simulink model "SG__MDL_IO104_VirtualShift"  (R2022a)
settings: Solver=FixedStepAuto  StartTime=0.0  StopTime=Inf  RelTol=1e-3  EnableMultiTasking=on
model workspace (MAT data in the model file):
  a = 0.28
  ff = 1200
  fi = 150
  tmax = 40
undefined symbols (not defined in the file or in its folder): Ended, Single
libraries: simulink x4, speedgoatlib_IO104 x3, hdlsllib x2, slrealtimeloglib x1, dspsrcs4 x1
settings Model: SimulationMode=external  Creator=padlewsk  LastModifiedBy=padlewsk
settings SolverCC: ConcurrentTasks=on  AlgebraicLoopSolver=TrustRegion  PositivePriorityOrder=on  AutoInsertRateTranBlk=on
settings DataIOCC: SaveFormat=StructureWithTime
settings OptimizationCC: BlockReduction=off  OptimizeBlockIOStorage=off
settings DebuggingCC: TasksWithSamePriorityMsg=none  UnconnectedInputMsg=warning  UnconnectedOutputMsg=warning  UnconnectedLineMsg=warning
settings HardwareCC: ProdBitPerLong=64  ProdLongLongMode=on  ProdHWDeviceType=Intel->x86-64 (Linux 64)
settings RTWCC: Description=Simulink Real-Time  SystemTargetFile=slrealtime.tlc  TemplateMakefile=slrealtime_default_tmf  Toolchain=Simulink Real-Time Toolchain  BuildConfiguration=Faster Runs  CodeExecutionProfiling=on  TargetLang=C++

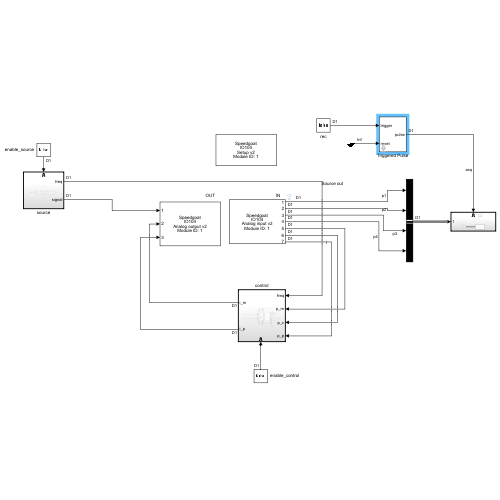
[thumbnail: Simulink's stored preview of the top-level diagram]
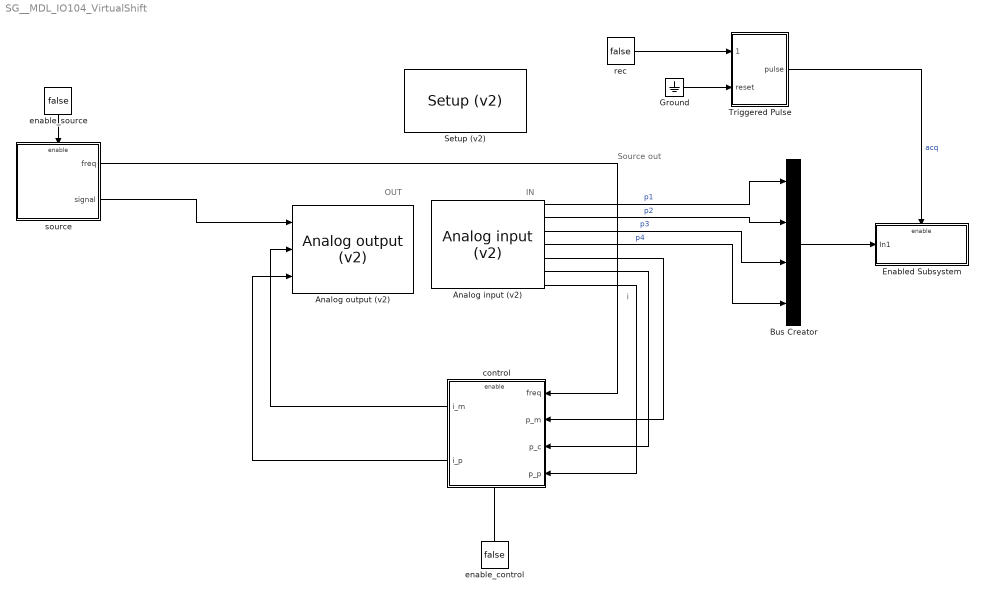
== system SG__MDL_IO104_VirtualShift ==
  note: i
  note: Source out
  note: IN
  note: OUT
  "Analog input (v2) " : speedgoatlib_IO104/Analog input (v2)   parModuleId=1  parTs=-1  parPciSlot=-1  parAdChannels=[1,2,3,4,5,6,7]  parAdChannelsSorted=[1,2,3,4,5,6,7]  parAdRange1=+-10V  parAdRange2=+-10V  parAdCoupling=Single-Ended  parAdFrameSize=1  parAdUseTrigger=off  parAdClockInitiator=Initiator  parAdSampleTime=9.920634921e-07  parTriggerInitiator=Target  parTriggerRate=4.161015625e-01
      settings: SourceProductName=Simulink Real-Time: Speedgoat I/O Blockset
  "Analog output (v2) " : speedgoatlib_IO104/Analog output (v2)   parModuleId=1  parTs=-1  parPciSlot=-1  parDaChannels=[1,2,3]  parDaChannelsSorted=[1,2,3]  parDaInitValue=[0,0,0]  parDaReset=[1,1,1]  parDaRange=+-10V  parDaFrameSize=1  parDaUseTrigger=off  parDaClockInitiator=Initiator  parDaSampleTime=9.920634921e-07  parTriggerInitiator=Target  parTriggerRate=4.161015625e-01  parAdBlockPresent=1
      settings: SourceProductName=Simulink Real-Time: Speedgoat I/O Blockset
  Bus Creator : BusCreator  Inputs=4
  Enabled Subsystem : Subsystem  TreatAsAtomicUnit=on
  Ground : Ground
  "Setup (v2) " : speedgoatlib_IO104/Setup (v2)   parPciSlot=-1  parModuleId=1  parTriggerInitiator=Target  parTriggerRate=4.161015625e-01  parCalibrate=on  parAdChannels=[1:7]  parAdRange1=+-10V  parAdRange2=+-10V  parAdCoupling=Single-Ended  parAdUseTrigger=off  parAdFrameSize=1  parAdClockInitiator=Initiator  parAdSampleTime=9.920634921e-07  parDaChannels=[1:3]  parDaChannelsSorted=[1,2,3]  parDaInitValue=[0]  parDaReset=[1]  parDaRange=+-10V  parDaUseTrigger=off  parDaFrameSize=1  parDaClockInitiator=Initiator  parDaSampleTime=9.920634921e-07  parDioByte0Dir=Outputs  parDioByte1Dir=Inputs  parDoChannels=[1:4]  parDoInitValues=[0]  parDoReset=[1]  parDiChannels=[13:16]
      settings: SourceProductName=Simulink Real-Time: Speedgoat I/O Blockset
  Triggered Pulse : Subsystem  mask(Triggered Pulse){N=4}
      mask prompts: N "Length (N samples)"
      mask help: Generates a single pulse of N samples length
  control : Subsystem
  enable_control : Constant  Value=false  SampleTime=-1
  enable_source : Constant  Value=false  SampleTime=-1
  rec : Constant  Value=false  SampleTime=-1
  source : Subsystem  TreatAsAtomicUnit=on
  wires:
  enable_source/1 -> source/Enable
  "Analog input (v2) "/3 -> Bus Creator/3  "p3"
  "Analog input (v2) "/1 -> Bus Creator/1  "p1"
  "Analog input (v2) "/2 -> Bus Creator/2  "p2"
  source/1(freq) -> control/1(freq)
  "Analog input (v2) "/5 -> control/2(p_m)
  control/2(i_p) -> "Analog output (v2) "/3
  enable_control/1 -> control/Enable
  "Analog input (v2) "/7 -> control/4(p_p)
  "Analog input (v2) "/6 -> control/3(p_c)
  source/2(signal) -> "Analog output (v2) "/1
  "Analog input (v2) "/4 -> Bus Creator/4  "p4"
  control/1(i_m) -> "Analog output (v2) "/2
  Triggered Pulse/1(pulse) -> Enabled Subsystem/Enable  "acq"
  Ground/1 -> Triggered Pulse/2(reset)
  rec/1 -> Triggered Pulse/1(trigger)
  Bus Creator/1 -> Enabled Subsystem/1(In1)

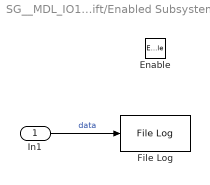
== system SG__MDL_IO104_VirtualShift/Enabled Subsystem ==
  In1 : Inport
  Enable : EnablePort
  File Log : slrealtimeloglib/File Log  decimation=1  inputProcessing=Elements as channels (sample based)
      settings: SourceProductBaseCode=XP
  wires:
  In1/1 -> File Log/1  "data"

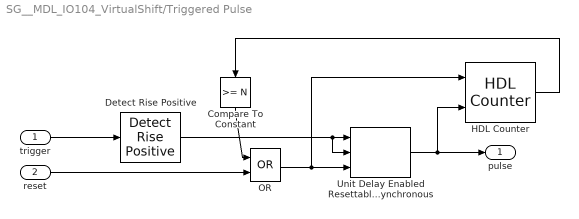
== system SG__MDL_IO104_VirtualShift/Triggered Pulse ==
  trigger : Inport
  reset : Inport  Port=2
  Compare To Constant : simulink/Logic and Bit Operations/Compare To Constant  relop=>=  const=N  OutDataTypeStr=boolean
  Detect Rise Positive : simulink/Logic and Bit Operations/Detect Rise Positive  vinit=0  OutDataTypeStr=boolean
  HDL Counter : hdlsllib/Sources/HDL Counter  CountType=Free running  CountInit=1  CountStep=1  CountMax=25  CountFromType=Initial value  CountFrom=1  CountResetPort=on  CountLoadPort=off  CountEnbPort=on  CountDirPort=off  CountHitOutputPort=off  CountDataType=Unsigned  CountWordLen=32  CountFracLen=0  CountSampTime=1
  OR : Logic  Operator=OR  AllPortsSameDT=off  OutDataTypeStr=boolean
  Unit Delay Enabled Resettable Synchronous : hdlsllib/Discrete/Unit Delay Enabled Resettable Synchronous  InitialCondition=0.0  SampleTime=-1
      settings: SourceProductBaseCode=SL
  pulse : Outport  VectorParamsAs1DForOutWhenUnconnected=off
  wires:
  OR/1 -> Unit Delay Enabled Resettable Synchronous/3, HDL Counter/1
  trigger/1 -> Detect Rise Positive/1
  Unit Delay Enabled Resettable Synchronous/1 -> HDL Counter/2, pulse/1
  Compare To Constant/1 -> OR/1
  reset/1 -> OR/2
  Detect Rise Positive/1 -> Unit Delay Enabled Resettable Synchronous/1, Unit Delay Enabled Resettable Synchronous/2
  HDL Counter/1 -> Compare To Constant/1

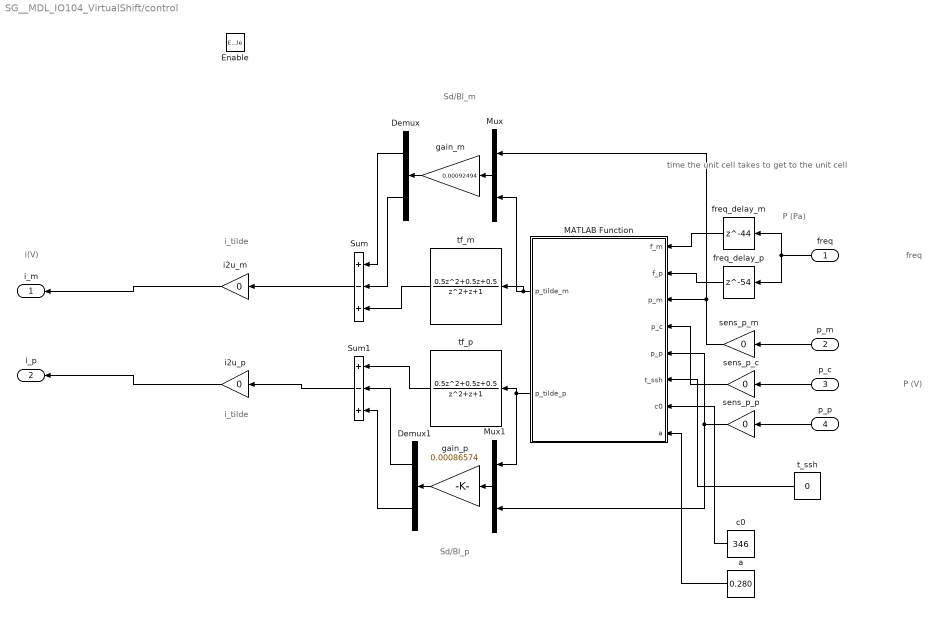
== system SG__MDL_IO104_VirtualShift/control ==
  note: time the unit cell takes to get to the unit cell
  note: Sd/Bl_p
  note: P (Pa)
  note: P (V)
  note: i_tilde
  note: i(V)
  note: freq
  note: i_tilde
  note: Sd/Bl_m
  freq : Inport
  p_m : Inport  Port=2
  p_c : Inport  Port=3
  p_p : Inport  Port=4
  Enable : EnablePort
  Demux : Demux  Outputs=2
  Demux1 : Demux  Outputs=2
  MATLAB Function : MATLAB Function  TreatAsAtomicUnit=on
  Mux : Mux  Inputs=2
  Mux1 : Mux  Inputs=2
  Sum : Sum  Inputs=+-+
  Sum1 : Sum  Inputs=+-+
  a : Constant  Value=0.280
  c0 : Constant  Value=346
  freq_delay_m : Delay  DelayLength=44  InitialCondition=1
  freq_delay_p : Delay  DelayLength=54  InitialCondition=1
  gain_m : Gain  Gain=0.00092494
  gain_p : Gain  Gain=0.00086574
  i2u_m : Gain  Gain=0
  i2u_p : Gain  Gain=0
  sens_p_c : Gain  Gain=0
  sens_p_m : Gain  Gain=0
  sens_p_p : Gain  Gain=0
  t_ssh : Constant  Value=0
  tf_m : DiscreteTransferFcn  Numerator="[0.5         0.5         0.5]"  Denominator="[1  1  1]"
  tf_p : DiscreteTransferFcn  Numerator="[0.5         0.5         0.5]"  Denominator="[1  1  1]"
  i_m : Outport
  i_p : Outport  Port=2
  wires:
  p_m/1 -> sens_p_m/1
  sens_p_m/1 -> Mux/1, MATLAB Function/3(p_m)
  p_c/1 -> sens_p_c/1
  p_p/1 -> sens_p_p/1
  t_ssh/1 -> MATLAB Function/6(t_ssh)
  sens_p_c/1 -> MATLAB Function/4(p_c)
  sens_p_p/1 -> MATLAB Function/5(p_p), Mux1/2
  Demux1/1 -> Sum1/2
  Demux1/2 -> Sum1/3
  Demux/2 -> Sum/2
  Demux/1 -> Sum/1
  Mux/1 -> gain_m/1
  gain_m/1 -> Demux/1
  Mux1/1 -> gain_p/1
  gain_p/1 -> Demux1/1
  tf_m/1 -> Sum/3
  tf_p/1 -> Sum1/1
  freq/1 -> freq_delay_p/1, freq_delay_m/1
  i2u_p/1 -> i_p/1
  freq_delay_m/1 -> MATLAB Function/1(f_m)
  i2u_m/1 -> i_m/1
  freq_delay_p/1 -> MATLAB Function/2(f_p)
  c0/1 -> MATLAB Function/7(c0)
  a/1 -> MATLAB Function/8(a)
  MATLAB Function/2(p_tilde_p) -> Mux1/1, tf_p/1
  MATLAB Function/1(p_tilde_m) -> tf_m/1, Mux/2
  Sum/1 -> i2u_m/1
  Sum1/1 -> i2u_p/1

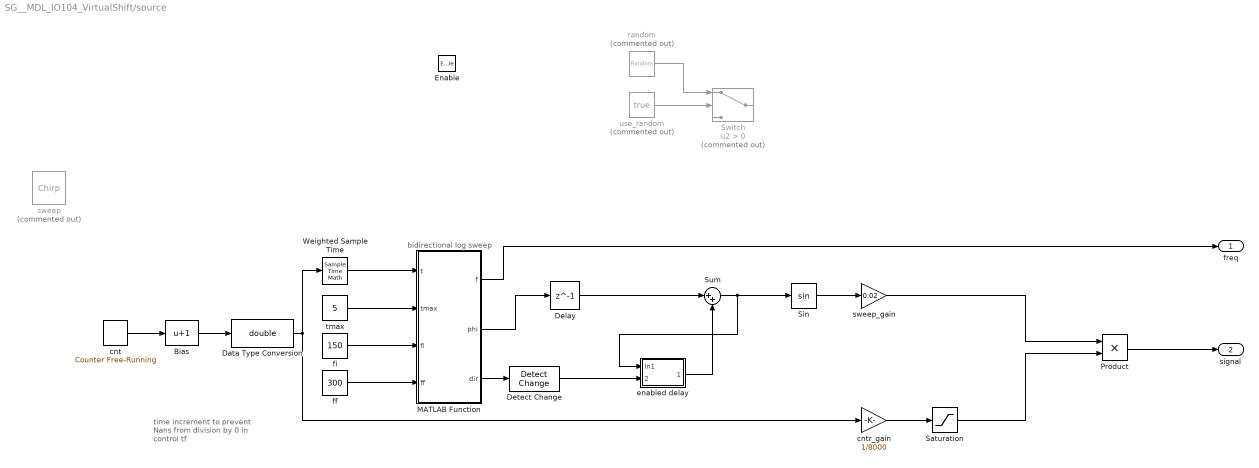
== system SG__MDL_IO104_VirtualShift/source ==
  note: bidirectional log sweep
  note: time increment to prevent Nans from division by 0 in control tf
  Enable : EnablePort  StatesWhenEnabling=reset
  Bias : Bias  Bias=1  SaturateOnIntegerOverflow=off
  Data Type Conversion : DataTypeConversion  OutDataTypeStr=double  SaturateOnIntegerOverflow=off  RndMeth=Floor
  Delay : Delay  DelayLength=1
  Detect Change : simulink/Logic and Bit Operations/Detect Change  vinit=false  OutDataTypeStr=boolean
  MATLAB Function : MATLAB Function  TreatAsAtomicUnit=on
  Product : Product
  Saturation : Saturate  UpperLimit=1  LowerLimit=0
  Sin : Trigonometry
  Sum : Sum  Inputs=|++
  Switch : Switch  Commented=on  Criteria=u2 > Threshold  SaturateOnIntegerOverflow=off  InputSameDT=off
  Weighted Sample Time : SampleTimeMath  TsampMathOp=*
  cnt : simulink/Sources/Counter Free-Running  NumBits=32  tsamp=4e-05
  cntr_gain : Gain  Gain=1/8000  ParamDataTypeStr=double
  enabled delay : Subsystem
  ff : Constant  Value=300
  fi : Constant  Value=150
  random : RandomNumber  Commented=on  Variance=0.5  SampleTime=3.5e-05
  sweep : dspsrcs4/Chirp  Commented=on  sweep=Logarithmic  mode=Bidirectional  f0=150  f1=1200  t1=10  Tsweep=20  phase=0  Ts=3.5e-05  spf=1  datatype=Double  OutputFrames=off
  sweep_gain : Gain  Gain=0.02
  tmax : Constant  Value=5
  use_random : Constant  Commented=on  Value=true  SampleTime=-1
  freq : Outport  OutputWhenDisabled=reset  InitialOutput=0  VectorParamsAs1DForOutWhenUnconnected=off
  signal : Outport  Port=2  OutputWhenDisabled=reset  InitialOutput=0  VectorParamsAs1DForOutWhenUnconnected=off
  wires:
  use_random/1 -> Switch/2
  random/1 -> Switch/1
  sweep_gain/1 -> Product/1
  cntr_gain/1 -> Saturation/1
  Product/1 -> signal/1
  MATLAB Function/2(phi) -> Delay/1
  Saturation/1 -> Product/2
  Weighted Sample Time/1 -> MATLAB Function/1(t)
  Data Type Conversion/1 -> cntr_gain/1, Weighted Sample Time/1
  MATLAB Function/1(f) -> freq/1
  Sin/1 -> sweep_gain/1
  MATLAB Function/3(dir) -> Detect Change/1
  Detect Change/1 -> enabled delay/2(enable)
  Delay/1 -> Sum/1
  enabled delay/1(Out1) -> Sum/2
  Sum/1 -> enabled delay/1(In1), Sin/1
  cnt/1 -> Bias/1
  Bias/1 -> Data Type Conversion/1
  ff/1 -> MATLAB Function/4(ff)
  tmax/1 -> MATLAB Function/2(tmax)
  fi/1 -> MATLAB Function/3(fi)

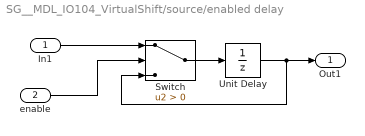
== system SG__MDL_IO104_VirtualShift/source/enabled delay ==
  In1 : Inport
  enable : Inport  Port=2
  Switch : Switch  Criteria=u2 > Threshold  SaturateOnIntegerOverflow=off  InputSameDT=off
  Unit Delay : UnitDelay  SampleTime=-1  HasFrameUpgradeWarning=on
  Out1 : Outport
  wires:
  Unit Delay/1 -> Switch/3, Out1/1
  Switch/1 -> Unit Delay/1
  In1/1 -> Switch/1
  enable/1 -> Switch/2

== matlab function SG__MDL_IO104_VirtualShift/control/MATLAB Function ==
  data: f_m input; f_p input; p_tilde_m output; p_m input; p_c input; p_p input; t_ssh input; p_tilde_p output; c0 input; a input
function [p_tilde_m, p_tilde_p] = p_tilde(f_m,f_p,p_m,p_c,p_p, t_ssh, c0, a)%frequency and pressure
% c0 and a are set as parameters and directly read from the workspace 
k_m = 2*pi*f_m/c0 %corresponding wave vector%%
k_p = 2*pi*f_p/c0 %corresponding wave vector%%

p_tilde_m = (p_m*sin(k_m*a*(t_ssh-1)/4) + p_c*sin(-k_m*a*t_ssh/4))/sin(-k_m*a/4) ;
p_tilde_p = (p_p*sin(-k_p*a*(t_ssh-1)/4) + p_c*sin(k_p*a*t_ssh/4))/sin(k_p*a/4) ;

%p_tilde_m = (p_c);
%p_tilde_p = (p_c);

== matlab function SG__MDL_IO104_VirtualShift/source/MATLAB Function ==
  data: f output; t input; tmax input; phi output; dir output; fi input; ff input
function [f, phi, dir] = fcn(t, tmax, fi, ff)
%tmax is the time at which the maximum frequency is reached

t = mod(t, 2*tmax);

if t < tmax
    % up
    dir = 1;
    
    
    % linear (CF wikipedia)
%     phi = 2*pi*(0.5*(ff - fi)*t^2/tmax + fi*t);
%     f = fi + (ff - fi)*t/tmax;
    
    % logarithmic %%% https://en.wikipedia.org/wiki/Chirp
    k = log((ff/fi)^(1/tmax));
    phi = 2*pi*fi*(exp(k*t) - 1)/k;
    f = fi*exp(k*t);
else
    % down
    dir = -1;
    
    
    % linear (CF wikipedia)
%     phi = 2*pi*(0.5*(fi - ff)*(t-tmax)^2/tmax + ff*(t-tmax)); % linear
%     f = ff + (fi - ff)*(t - tmax)/tmax;
    
    % logarithmic
    k = log((fi/ff)^(1/tmax));
    phi = 2*pi*ff*(exp(k*(t - tmax)) - 1)/k;
    f = ff*exp(k*(t-tmax));
end

phi = mod(phi, 2*pi);
